simulink model "Clase_6"  (R2021a)
settings: Solver=VariableStepAuto  StartTime=0.0  StopTime=5  MaxStep=0.001  RelTol=1e-4
libraries: cstblocks x2
settings Model: Creator=nicoh  LastModifiedBy=nicoh

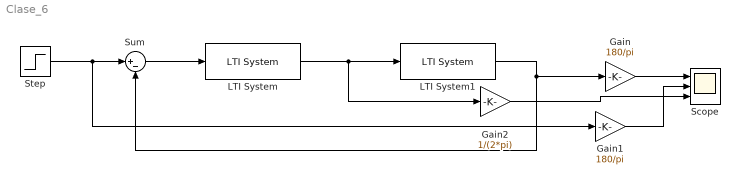
== system Clase_6 ==
  Gain : Gain  Gain=180/pi
  Gain1 : Gain  Gain=180/pi
  Gain2 : Gain  Gain=1/(2*pi)
  LTI System : cstblocks/LTI System  sys=C_pid  IC=[]
  LTI System1 : cstblocks/LTI System  sys=P  IC=[]
  Scope : Scope  NumInputPorts=3
  Step : Step  Time=0.02  Before=5*(pi/180)  After=0  SampleTime=0
  Sum : Sum  Inputs=|+-
  wires:
  LTI System/1 -> Gain2/1, LTI System1/1
  Sum/1 -> LTI System/1
  Step/1 -> Gain1/1, Sum/1
  LTI System1/1 -> Gain/1, Sum/2
  Gain/1 -> Scope/1
  Gain1/1 -> Scope/2
  Gain2/1 -> Scope/3
